simulink model "MultiInstanceModelExample"  (Simulink 10.0)
settings: Solver=FixedStepDiscrete  StartTime=0.0  StopTime=20  FixedStep=0.1  RelTol=1e-3
settings Model: Creator=The MathWorks, Inc.  ModifiedByFormat=The MathWorks Inc.  LastModifiedBy=The MathWorks Inc.  ExtModeAutoUpdateStatusClock=off
settings DataIOCC: SaveFormat=StructureWithTime  SaveOutput=off  DSMLogging=off  InspectSignalLogs=on  SaveTime=off  SignalLoggingName=logsOut
settings OptimizationCC: DefaultParameterBehavior=Inlined  InlineInvariantSignals=on  ExpressionDepthLimit=2147483647  InitFltsAndDblsToZero=on
settings DebuggingCC: SaveWithParameterizedLinksMsg=none  UnderspecifiedInitializationDetection=Simplified  MergeDetectMultiDrivingBlocksExec=error  CheckExecutionContextPreStartOutputMsg=on  CheckExecutionContextRuntimeOutputMsg=on  MultiTaskDSMMsg=warning  MultiTaskCondExecSysMsg=none  SigSpecEnsureSampleTimeMsg=none  FcnCallInpInsideContextMsg=warning  AllowSymbolicDim=off  StateNameClashWarn=warning  StrictBusMsg=ErrorOnBusTreatedAsVector
settings HardwareCC: TargetHWDeviceType=32-bit Generic
settings ModelReferenceCC: UpdateModelReferenceTargets=IfOutOfDate  CheckModelReferenceTargetMessage=none
settings RTWCC: GenerateReport=on  LaunchReport=on
settings CodeAppCC: MaxIdLength=100
settings GRTTargetCC: TargetFcnLib=ansi_tfl_tmw.mat  GeneratePreprocessorConditionals=Disable all
settings ConfigComp: CovExternalEMLEnable=off  CovSFcnEnable=off

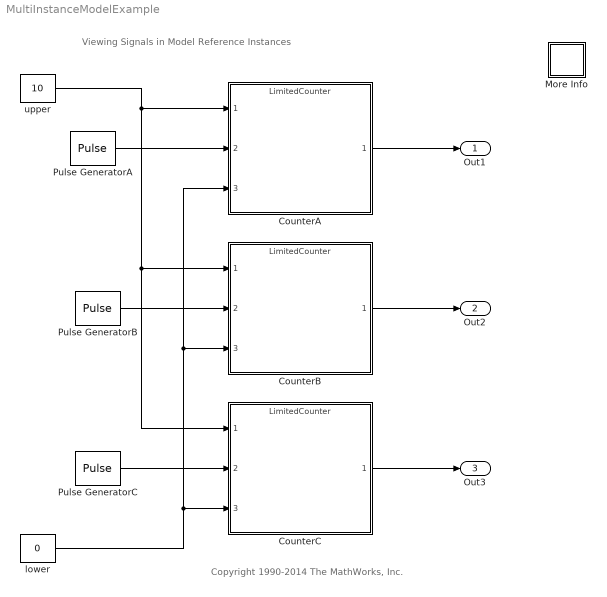
== system MultiInstanceModelExample ==
  note: Viewing Signals in Model Reference Instances
  note: Copyright 1990-2014 The MathWorks, Inc.
  CounterA : ModelReference  ModelNameDialog=LimitedCounter  SimulationMode=Normal  ModelReferenceVersion=1.89
  CounterB : ModelReference  DialogController=Simulink.DDGSource  ModelNameDialog=LimitedCounter  SimulationMode=Normal  ModelReferenceVersion=1.89
  CounterC : ModelReference  ModelNameDialog=LimitedCounter  ModelReferenceVersion=1.89
  More Info : Subsystem
      settings: OpenFcn=helpview(fullfile(docroot,'simulink','helptargets.map'), 'slexMultiInstanceMdlRefSignalInspectorScript');
      mask Display: disp('?')
  Pulse GeneratorA : DiscretePulseGenerator  SampleTime=0.1  VectorParams1D=off
      settings: AttributesFormatString=with Ts = %<SampleTime>
  Pulse GeneratorB : DiscretePulseGenerator  SampleTime=0.5  VectorParams1D=off
      settings: AttributesFormatString=with Ts = %<SampleTime>
  Pulse GeneratorC : DiscretePulseGenerator  SampleTime=1.0  VectorParams1D=off
      settings: AttributesFormatString=with Ts = %<SampleTime>
  lower : Constant  Value=0
  upper : Constant  Value=10
  Out1 : Outport  VectorParamsAs1DForOutWhenUnconnected=off
  Out2 : Outport  Port=2  VectorParamsAs1DForOutWhenUnconnected=off
  Out3 : Outport  Port=3  VectorParamsAs1DForOutWhenUnconnected=off
  wires:
  Pulse GeneratorA/1 -> CounterA/2
  Pulse GeneratorB/1 -> CounterB/2
  Pulse GeneratorC/1 -> CounterC/2
  lower/1 -> CounterA/3, CounterB/3, CounterC/3
  upper/1 -> CounterC/1, CounterB/1, CounterA/1
  CounterA/1 -> Out1/1
  CounterB/1 -> Out2/1
  CounterC/1 -> Out3/1

== system MultiInstanceModelExample/More Info ==
  note: Bus Block Demonstration
  note: This demonstration shows how signals may be grouped and ungrouped while
      | retaining their names.  In this demonstration, 5 signals are created and labelled
      | appropriately.  These signals are then mux'd together to create a bus of signals.
      | This bus of signals is then fed into the Bus Selector block.  Inside of the Bus
      | Selector block, the Pulse and Chirp signals are chosen to be output from the
      | original signal bus.
      |
      | It is possible to place a nest signal buses and then still retrieve the original signal
      | with its label.
